simulink model "model1"  (R2020b)
settings: Solver=FixedStepAuto  StartTime=0.0  StopTime=10.0  RelTol=1e-3
libraries: simulink x2, hdlsllib x1
settings Model: Creator=pablo  LastModifiedBy=pablo
settings DebuggingCC: AlgebraicLoopMsg=error
settings HardwareCC: ProdBitPerPointer=32  ProdBitPerSizeT=32  ProdBitPerPtrDiffT=32  ProdLargestAtomicFloat=None  ProdIntDivRoundTo=Undefined  ProdEndianess=Unspecified  ProdWordSize=32  ProdHWDeviceType=ASIC/FPGA->ASIC/FPGA  TargetBitPerLong=64  TargetBitPerPointer=64  TargetBitPerSizeT=64  TargetBitPerPtrDiffT=64  TargetLongLongMode=on  TargetIntDivRoundTo=Zero  TargetEndianess=LittleEndian  TargetWordSize=64  TargetHWDeviceType=Custom Processor->MATLAB Host Computer  ProdEqTarget=off

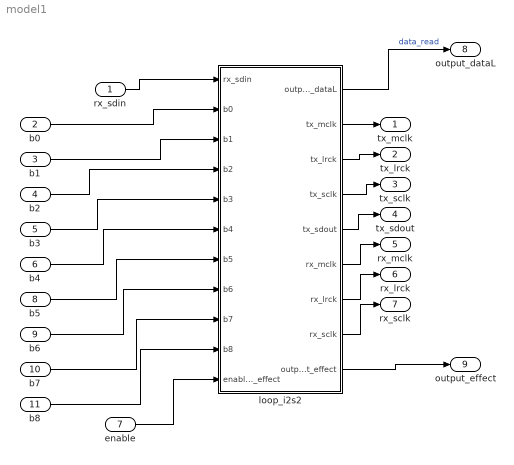
== system model1 ==
  rx_sdin : Inport
  b0 : Inport  Port=2  OutDataTypeStr=int32
  b1 : Inport  Port=3  OutDataTypeStr=int32
  b2 : Inport  Port=4  OutDataTypeStr=int32
  b3 : Inport  Port=5  OutDataTypeStr=int32
  b4 : Inport  Port=6  OutDataTypeStr=int32
  enable : Inport  Port=7  OutDataTypeStr=int32
  b5 : Inport  Port=8  OutDataTypeStr=int32
  b6 : Inport  Port=9  OutDataTypeStr=int32
  b7 : Inport  Port=10  OutDataTypeStr=int32
  b8 : Inport  Port=11  OutDataTypeStr=int32
  loop_i2s2 : Subsystem  TreatAsAtomicUnit=on
  tx_mclk : Outport  VectorParamsAs1DForOutWhenUnconnected=off
  tx_lrck : Outport  Port=2  VectorParamsAs1DForOutWhenUnconnected=off
  tx_sclk : Outport  Port=3  VectorParamsAs1DForOutWhenUnconnected=off
  tx_sdout : Outport  Port=4  VectorParamsAs1DForOutWhenUnconnected=off
  rx_mclk : Outport  Port=5  VectorParamsAs1DForOutWhenUnconnected=off
  rx_lrck : Outport  Port=6  VectorParamsAs1DForOutWhenUnconnected=off
  rx_sclk : Outport  Port=7  VectorParamsAs1DForOutWhenUnconnected=off
  output_dataL : Outport  Port=8  OutDataTypeStr=fixdt(1,24,23)  VectorParamsAs1DForOutWhenUnconnected=off
  output_effect : Outport  Port=9  OutDataTypeStr=fixdt(1,24,23)  VectorParamsAs1DForOutWhenUnconnected=off
  wires:
  loop_i2s2/1(output_dataL) -> output_dataL/1  "data_read"
  rx_sdin/1 -> loop_i2s2/1(rx_sdin)
  loop_i2s2/2(tx_mclk) -> tx_mclk/1
  loop_i2s2/3(tx_lrck) -> tx_lrck/1
  loop_i2s2/4(tx_sclk) -> tx_sclk/1
  loop_i2s2/5(tx_sdout) -> tx_sdout/1
  loop_i2s2/6(rx_mclk) -> rx_mclk/1
  loop_i2s2/7(rx_lrck) -> rx_lrck/1
  loop_i2s2/8(rx_sclk) -> rx_sclk/1
  b0/1 -> loop_i2s2/2(b0)
  b1/1 -> loop_i2s2/3(b1)
  b2/1 -> loop_i2s2/4(b2)
  b3/1 -> loop_i2s2/5(b3)
  b4/1 -> loop_i2s2/6(b4)
  enable/1 -> loop_i2s2/11(enable_effect)
  loop_i2s2/9(output_effect) -> output_effect/1
  b5/1 -> loop_i2s2/7(b5)
  b6/1 -> loop_i2s2/8(b6)
  b7/1 -> loop_i2s2/9(b7)
  b8/1 -> loop_i2s2/10(b8)

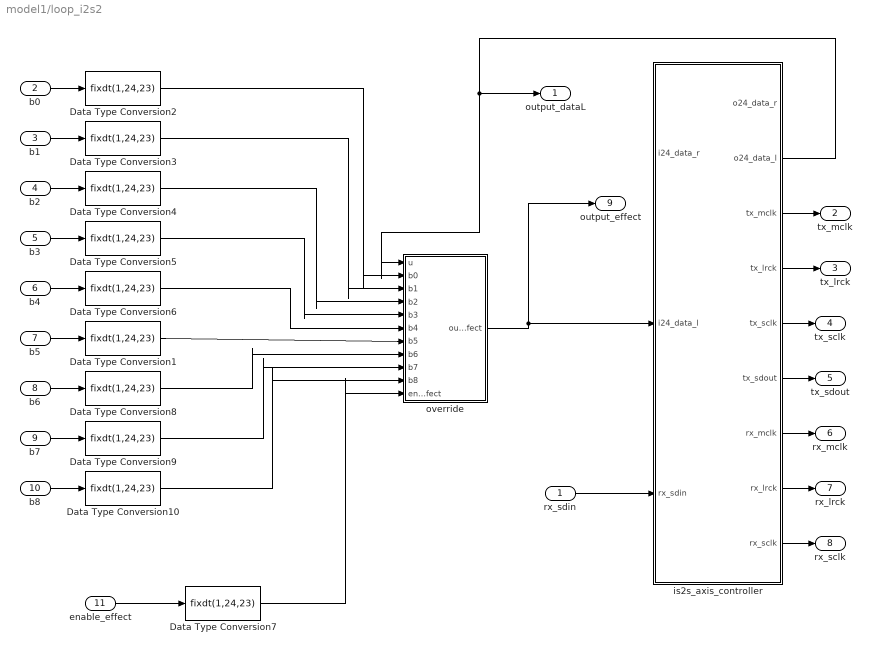
== system model1/loop_i2s2 ==
  rx_sdin : Inport  OutDataTypeStr=boolean
  b0 : Inport  Port=2  OutDataTypeStr=int32
  b1 : Inport  Port=3  OutDataTypeStr=int32
  b2 : Inport  Port=4  OutDataTypeStr=int32
  b3 : Inport  Port=5  OutDataTypeStr=int32
  b4 : Inport  Port=6  OutDataTypeStr=int32
  b5 : Inport  Port=7  OutDataTypeStr=int32
  b6 : Inport  Port=8  OutDataTypeStr=int32
  b7 : Inport  Port=9  OutDataTypeStr=int32
  b8 : Inport  Port=10  OutDataTypeStr=int32
  enable_effect : Inport  Port=11  OutDataTypeStr=int32
  Data Type Conversion{1..10} (10 alike) : DataTypeConversion  OutDataTypeStr=fixdt(1,24,23)
  is2s_axis_controller : Subsystem
  override : Subsystem
  output_dataL : Outport  OutDataTypeStr=fixdt(1,24,23)
  tx_mclk : Outport  Port=2  VectorParamsAs1DForOutWhenUnconnected=off
  tx_lrck : Outport  Port=3  VectorParamsAs1DForOutWhenUnconnected=off
  tx_sclk : Outport  Port=4  VectorParamsAs1DForOutWhenUnconnected=off
  tx_sdout : Outport  Port=5  VectorParamsAs1DForOutWhenUnconnected=off
  rx_mclk : Outport  Port=6  VectorParamsAs1DForOutWhenUnconnected=off
  rx_lrck : Outport  Port=7  VectorParamsAs1DForOutWhenUnconnected=off
  rx_sclk : Outport  Port=8  VectorParamsAs1DForOutWhenUnconnected=off
  output_effect : Outport  Port=9  OutDataTypeStr=fixdt(1,24,23)
  wires:
  is2s_axis_controller/3(tx_mclk) -> tx_mclk/1
  is2s_axis_controller/4(tx_lrck) -> tx_lrck/1
  is2s_axis_controller/5(tx_sclk) -> tx_sclk/1
  is2s_axis_controller/6(tx_sdout) -> tx_sdout/1
  is2s_axis_controller/7(rx_mclk) -> rx_mclk/1
  is2s_axis_controller/8(rx_lrck) -> rx_lrck/1
  is2s_axis_controller/9(rx_sclk) -> rx_sclk/1
  rx_sdin/1 -> is2s_axis_controller/3(rx_sdin)
  b0/1 -> Data Type Conversion2/1
  b1/1 -> Data Type Conversion3/1
  b2/1 -> Data Type Conversion4/1
  b3/1 -> Data Type Conversion5/1
  b4/1 -> Data Type Conversion6/1
  enable_effect/1 -> Data Type Conversion7/1
  override/1(output_effect) -> is2s_axis_controller/2(i24_data_l), output_effect/1
  is2s_axis_controller/2(o24_data_l) -> output_dataL/1, override/1(u)
  Data Type Conversion2/1 -> override/2(b0)
  Data Type Conversion3/1 -> override/3(b1)
  Data Type Conversion4/1 -> override/4(b2)
  Data Type Conversion5/1 -> override/5(b3)
  Data Type Conversion6/1 -> override/6(b4)
  Data Type Conversion7/1 -> override/11(enable_effect)
  b5/1 -> Data Type Conversion1/1
  b6/1 -> Data Type Conversion8/1
  b7/1 -> Data Type Conversion9/1
  b8/1 -> Data Type Conversion10/1
  Data Type Conversion1/1 -> override/7(b5)
  Data Type Conversion8/1 -> override/8(b6)
  Data Type Conversion9/1 -> override/9(b7)
  Data Type Conversion10/1 -> override/10(b8)

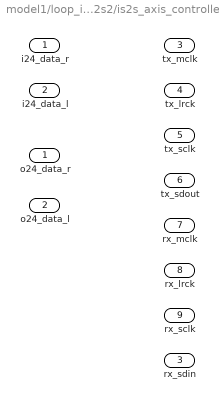
== system model1/loop_i2s2/is2s_axis_controller ==
  i24_data_r : Inport  OutDataTypeStr=fixdt(1,24,23)
  i24_data_l : Inport  Port=2  OutDataTypeStr=fixdt(1,24,23)
  rx_sdin : Inport  Port=3
  o24_data_r : Outport  OutDataTypeStr=fixdt(1,24,23)
  o24_data_l : Outport  Port=2  OutDataTypeStr=fixdt(1,24,23)
  tx_mclk : Outport  Port=3  OutDataTypeStr=boolean
  tx_lrck : Outport  Port=4  OutDataTypeStr=boolean
  tx_sclk : Outport  Port=5  OutDataTypeStr=boolean
  tx_sdout : Outport  Port=6  OutDataTypeStr=boolean
  rx_mclk : Outport  Port=7  OutDataTypeStr=boolean
  rx_lrck : Outport  Port=8  OutDataTypeStr=boolean
  rx_sclk : Outport  Port=9  OutDataTypeStr=boolean

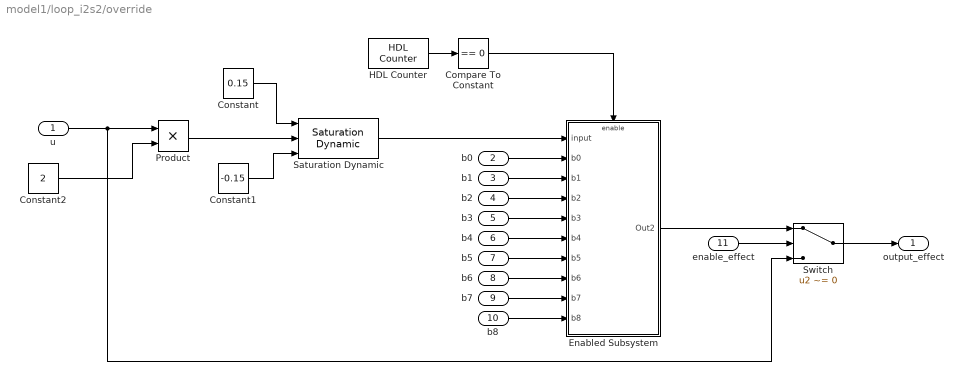
== system model1/loop_i2s2/override ==
  u : Inport  OutDataTypeStr=fixdt(1,24,23)
  b0 : Inport  Port=2  OutDataTypeStr=fixdt(1,24,23)
  b1 : Inport  Port=3  OutDataTypeStr=fixdt(1,24,23)
  b2 : Inport  Port=4  OutDataTypeStr=fixdt(1,24,23)
  b3 : Inport  Port=5  OutDataTypeStr=fixdt(1,24,23)
  b4 : Inport  Port=6  OutDataTypeStr=fixdt(1,24,23)
  b5 : Inport  Port=7  OutDataTypeStr=fixdt(1,24,23)
  b6 : Inport  Port=8  OutDataTypeStr=fixdt(1,24,23)
  b7 : Inport  Port=9  OutDataTypeStr=fixdt(1,24,23)
  b8 : Inport  Port=10  OutDataTypeStr=fixdt(1,24,23)
  enable_effect : Inport  Port=11  OutDataTypeStr=fixdt(1,24,23)
  Compare To Constant : simulink/Logic and Bit Operations/Compare To Constant  relop===  const=0  OutDataTypeStr=boolean
  Constant : Constant  Value=0.15  OutDataTypeStr=fixdt(1,24,23)
  Constant1 : Constant  Value=-0.15  OutDataTypeStr=fixdt(1,24,23)
  Constant2 : Constant  Value=2  OutDataTypeStr=fixdt(1,25,23)
  Enabled Subsystem : Subsystem  TreatAsAtomicUnit=on
  HDL Counter : hdlsllib/Sources/HDL Counter  CountType=Free running  CountInit=0  CountStep=1  CountMax=25  CountFromType=Initial value  CountFrom=0  CountResetPort=off  CountLoadPort=off  CountEnbPort=off  CountDirPort=off  CountDataType=Unsigned  CountWordLen=9  CountFracLen=0  CountSampTime=1
  Product : Product  OutDataTypeStr=fixdt(1,24,23)
  Saturation Dynamic : simulink/Discontinuities/Saturation Dynamic  OutMin=[]  OutMax=[]  OutDataTypeStr=fixdt(1,24,23)  OutputDataTypeScalingMode=Specify via dialog  OutDataType=fixdt(1,24,23)  OutScaling=[]  DoSatur=off
  Switch : Switch  Criteria=u2 ~= 0  Threshold=0.5  OutDataTypeStr=fixdt(1,24,23)
  output_effect : Outport  OutDataTypeStr=fixdt(1,24,23)
  wires:
  b0/1 -> Enabled Subsystem/2(b0)
  b1/1 -> Enabled Subsystem/3(b1)
  b3/1 -> Enabled Subsystem/5(b3)
  b2/1 -> Enabled Subsystem/4(b2)
  b4/1 -> Enabled Subsystem/6(b4)
  u/1 -> Switch/3, Product/1
  Product/1 -> Saturation Dynamic/2
  enable_effect/1 -> Switch/2
  Switch/1 -> output_effect/1
  Constant/1 -> Saturation Dynamic/1
  Constant1/1 -> Saturation Dynamic/3
  Constant2/1 -> Product/2
  Enabled Subsystem/1(Out2) -> Switch/1
  b5/1 -> Enabled Subsystem/7(b5)
  b6/1 -> Enabled Subsystem/8(b6)
  b7/1 -> Enabled Subsystem/9(b7)
  b8/1 -> Enabled Subsystem/10(b8)
  Saturation Dynamic/1 -> Enabled Subsystem/1(input)
  HDL Counter/1 -> Compare To Constant/1
  Compare To Constant/1 -> Enabled Subsystem/Enable

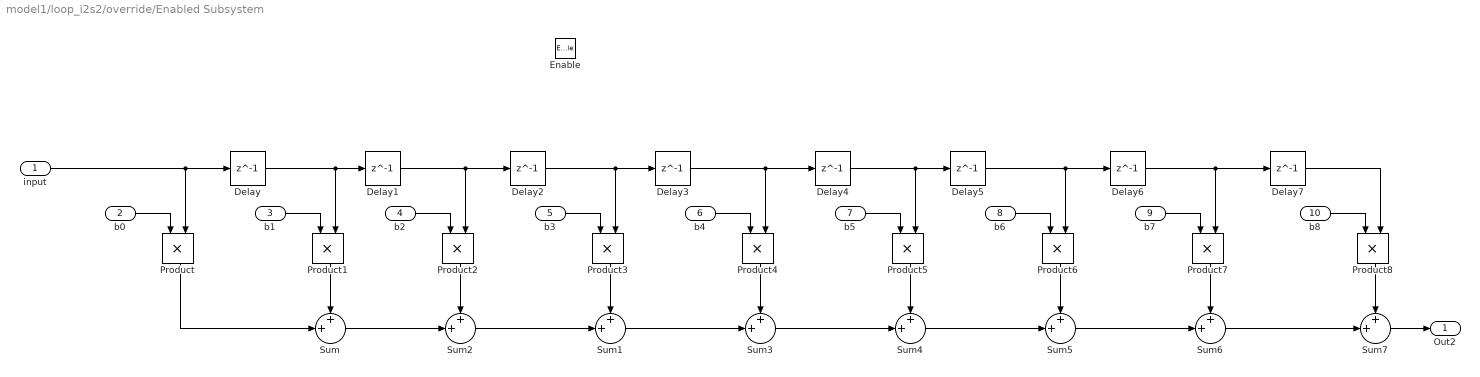
== system model1/loop_i2s2/override/Enabled Subsystem ==
  input : Inport  OutDataTypeStr=fixdt(1,24,23)
  b0 : Inport  Port=2  OutDataTypeStr=fixdt(1,24,23)
  b1 : Inport  Port=3  OutDataTypeStr=fixdt(1,24,23)
  b2 : Inport  Port=4  OutDataTypeStr=fixdt(1,24,23)
  b3 : Inport  Port=5  OutDataTypeStr=fixdt(1,24,23)
  b4 : Inport  Port=6  OutDataTypeStr=fixdt(1,24,23)
  b5 : Inport  Port=7  OutDataTypeStr=fixdt(1,24,23)
  b6 : Inport  Port=8  OutDataTypeStr=fixdt(1,24,23)
  b7 : Inport  Port=9  OutDataTypeStr=fixdt(1,24,23)
  b8 : Inport  Port=10  OutDataTypeStr=fixdt(1,24,23)
  Enable : EnablePort  PropagateVarSize=During execution
  Delay{,1..7} (8 alike) : Delay  DelayLength=1  InitialCondition=0
  Product{,1..8} (9 alike) : Product  OutDataTypeStr=fixdt(1,24,23)
  Sum : Sum  Inputs=++|  OutDataTypeStr=fixdt(1,32,31)
  Sum{1..3,5..7} (6 alike) : Sum  Inputs=++|  OutDataTypeStr=fixdt(1,24,23)
  Sum4 : Sum  Inputs=++|  AccumDataTypeStr=fixdt(1,24,23)  OutDataTypeStr=fixdt(1,24,23)
  Out2 : Outport  OutDataTypeStr=fixdt(1,24,23)  InitialOutput=0
  wires:
  Sum1/1 -> Sum3/2
  Sum4/1 -> Sum5/2
  b6/1 -> Product6/1
  Product1/1 -> Sum/1
  b7/1 -> Product7/1
  b5/1 -> Product5/1
  Delay7/1 -> Product8/2
  b4/1 -> Product4/1
  b2/1 -> Product2/1
  Delay3/1 -> Delay4/1, Product4/2
  Delay1/1 -> Product2/2, Delay2/1
  Delay6/1 -> Delay7/1, Product7/2
  Product2/1 -> Sum2/1
  Product5/1 -> Sum4/1
  Product7/1 -> Sum6/1
  Delay5/1 -> Delay6/1, Product6/2
  Sum6/1 -> Sum7/2
  Product6/1 -> Sum5/1
  Sum2/1 -> Sum1/2
  Delay4/1 -> Delay5/1, Product5/2
  b1/1 -> Product1/1
  Product8/1 -> Sum7/1
  b0/1 -> Product/1
  Sum5/1 -> Sum6/2
  Product/1 -> Sum/2
  input/1 -> Delay/1, Product/2
  Delay2/1 -> Delay3/1, Product3/2
  Product4/1 -> Sum3/1
  Sum7/1 -> Out2/1
  Delay/1 -> Delay1/1, Product1/2
  Sum/1 -> Sum2/2
  Sum3/1 -> Sum4/2
  b3/1 -> Product3/1
  Product3/1 -> Sum1/1
  b8/1 -> Product8/1
